simulink model "parcial2022_planta"  (R2023a)
settings: Solver=VariableStepAuto  StartTime=0.0  StopTime=70  RelTol=1e-3
values from neighbouring files (symbols this model uses):
  b1 = 10e3    (= 10000)    [parcial2022.m]    (also in parcial2023.m = 1500; parcial2024.m = 625)
  b2 = 1e3    (= 1000)    [parcial2022.m]
  k1 = 1    [final2023_02_23.m]    (also in final2024.m = 1.2; parcial2022.m = 40000; parcial2023.m = 958; parcial2024.m = 1000)
  k2 = 19.8    [final2023_02_23.m]    (also in final2024.m = 1.3; parcial2022.m = 10000; parcial2023.m = 4410; parcial2024.m = 1500)
  m = 0.65    [final2023_02_23.m]    (also in parcial2022.m = 50000; parcial2025.m = 50)
  v0 = 200/9    (= 22.2222222222)    [parcial2022.m]
settings Model: Creator=Agustin  LastModifiedBy=Agustin

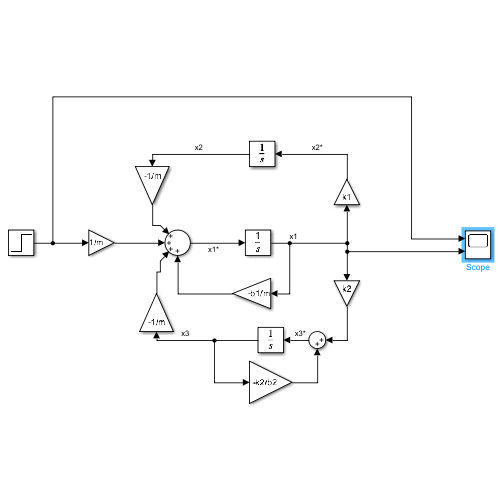
[thumbnail: Simulink's stored preview of the top-level diagram]
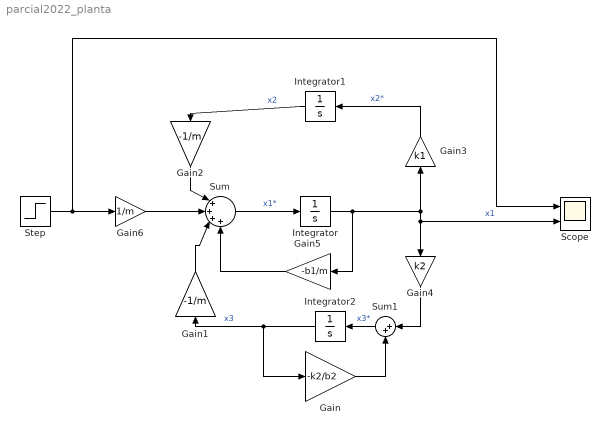
== system parcial2022_planta ==
  Gain : Gain  Gain=-k2/b2
  Gain1 : Gain  Gain=-1/m
  Gain2 : Gain  Gain=-1/m
  Gain3 : Gain  Gain=k1
  Gain4 : Gain  Gain=k2
  Gain5 : Gain  Gain=-b1/m
  Gain6 : Gain  Gain=1/m
  Integrator : Integrator  InitialCondition=v0
  Integrator1 : Integrator
  Integrator2 : Integrator
  Scope : Scope  NumInputPorts=2
  Step : Step  After=0  SampleTime=0
  Sum : Sum  Inputs=|++++
  Sum1 : Sum  Inputs=|++
  wires:
  Gain/1 -> Sum1/2
  Sum1/1 -> Integrator2/1  "x3*"
  Gain3/1 -> Integrator1/1  "x2*"
  Integrator1/1 -> Gain2/1  "x2"
  Gain2/1 -> Sum/1
  Gain1/1 -> Sum/3
  Step/1 -> Gain6/1, Scope/1
  Integrator2/1 -> Gain/1, Gain1/1  "x3"
  Sum/1 -> Integrator/1  "x1*"
  Integrator/1 -> Gain5/1, Gain4/1, Scope/2, Gain3/1  "x1"
  Gain4/1 -> Sum1/1
  Gain5/1 -> Sum/4
  Gain6/1 -> Sum/2
